simulink model "untitled"  (R2013a)
settings: Solver=ode45  StartTime=0.0  StopTime=20  RelTol=1e-3
settings Model: Creator=Sion  LastModifiedBy=Sion

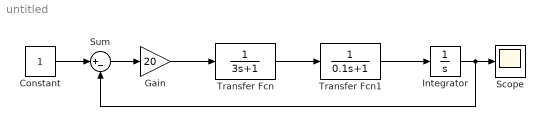
== system untitled ==
  Constant : Constant
  Gain : Gain  Gain=20
  Integrator : Integrator
  Scope : Scope
      settings: SaveName=ScopeData36
  Sum : Sum  Inputs=|+-
  Transfer Fcn : TransferFcn  Denominator=[3 1]
  Transfer Fcn1 : TransferFcn  Denominator=[0.1 1]
  wires:
  Integrator/1 -> Sum/2, Scope/1
  Transfer Fcn1/1 -> Integrator/1
  Transfer Fcn/1 -> Transfer Fcn1/1
  Gain/1 -> Transfer Fcn/1
  Sum/1 -> Gain/1
  Constant/1 -> Sum/1
